simulink model "Part_B"  (R2022b)
settings: Solver=VariableStepAuto  StartTime=0.0  StopTime=10.0  RelTol=1e-3
undefined symbols (not defined in the file): Ac, fc, Ka, sample_time
settings Model: Creator=DELL  LastModifiedBy=DELL

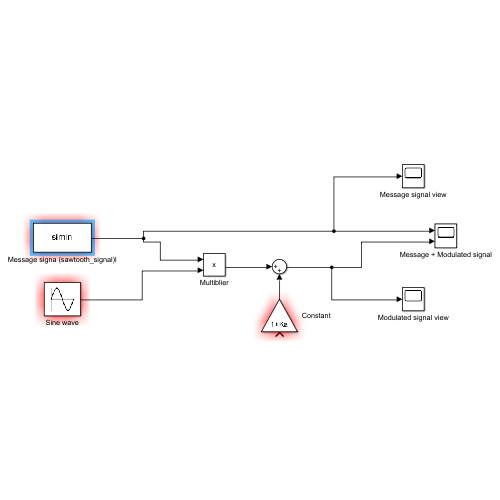
[thumbnail: Simulink's stored preview of the top-level diagram]
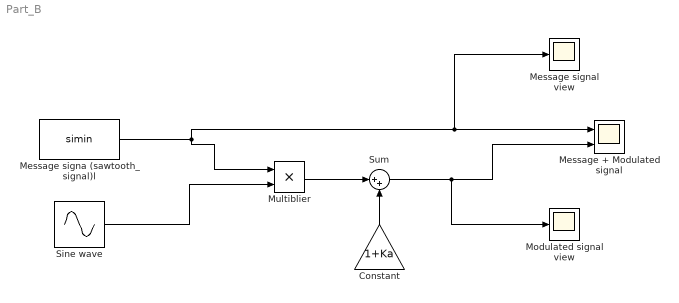
== system Part_B ==
  Constant : Gain  Gain=1+Ka
  Message + Modulated signal : Scope  NumInputPorts=2
  Message signa (sawtooth_signal)l : FromWorkspace  VariableName=simin  SampleTime=sample_time
  Message signal view : Scope
  Modulated signal view : Scope
  Multiblier : Product
  Sine wave : Sin  Amplitude=Ac  Frequency=fc  SampleTime=0
  Sum : Sum  Inputs=|++
  wires:
  Sine wave/1 -> Multiblier/2
  Multiblier/1 -> Sum/1
  Sum/1 -> Modulated signal view/1, Message + Modulated signal/2
  Message signa (sawtooth_signal)l/1 -> Multiblier/1, Message signal view/1, Message + Modulated signal/1
  Constant/1 -> Sum/2
